simulink model "balancing"  (Simulink 9.1)
settings: Solver=ode1  StartTime=0.0  StopTime=30  FixedStep=0.001  RelTol=1e-8  EnableMultiTasking=on
values from neighbouring files (symbols this model uses):
  A = [0  0    1    0 ... (first row only)    [parameters.m]    (also in parameters_real.m)
  B = (Km/Rm)*B    [parameters.m]    (also in parameters_real.m)
  C = [ 1 0 0 0 ... (first row only)    [parameters.m]    (also in parameters_real.m)
  E0 = 0.05    [parameters.m]    (also in parameters_real.m)
  g = 9.81    [parameters.m]    (also in parameters_real.m)
  J2cap = J2 + m2*(l2^2)    (= 0.0055028)    [parameters.m]    (also in parameters_real.m = 0.006520161)
  K = -lqr(A,B,Q,R)    [parameters.m]    (also in parameters_real.m)
  Km = 0.090    (= 0.09)    [parameters.m]    (also in parameters_real.m)
  l2 = 0.148    [parameters.m]    (also in parameters_real.m = 0.233)
  Lm = 0.005    [parameters.m]    (also in parameters_real.m)
  m2 = 0.075    [parameters.m]    (also in parameters_real.m = 0.049)
  Rm = 7.80    (= 7.8)    [parameters.m]    (also in parameters_real.m)
  w1 = J0cap*J2cap    (= 0.00020550921964)    [parameters.m]    (also in parameters_real.m = J0cap*J2cap)
  w2 = J2cap^2    (= 3.028080784e-05)    [parameters.m]    (also in parameters_real.m = 4.25124994659e-05)
  w3 = -(m2^2)*(L1^2)*(l2^2)    (= -9.52216164e-06)    [parameters.m]    (also in parameters_real.m = -4.08366901448e-06)
  x1 = (-J2cap * b1)    (= -5.5028e-07)    [parameters.m]    (also in parameters_real.m = -6.520161e-07)
  x2 = (m2* L1* l2* b2)    (= 8.64024e-07)    [parameters.m]    (also in parameters_real.m = 5.6582652e-07)
  x3 = - J2cap^2    (= -3.028080784e-05)    [parameters.m]    (also in parameters_real.m = -4.25124994659e-05)
  x4 = - 0.5 *J2cap *m2 *L1* l2    (= -8.49027012e-06)    [parameters.m]    (also in parameters_real.m = -6.58800001512e-06)
  x5 = J2cap *m2*L1*l2    (= 1.698054024e-05)    [parameters.m]    (also in parameters_real.m = 1.31760000302e-05)
  x6 = J2cap    (= 0.0055028)    [parameters.m]    (also in parameters_real.m = 0.006520161)
  x7 = -m2*L1*l2    (= -0.0030858)    [parameters.m]    (also in parameters_real.m = -0.002020809)
  x8 = 0.5* (m2^2)*(L1)*(l2^2)    (= 1.712619e-05)    [parameters.m]    (also in parameters_real.m = 1.15357881765e-05)
  y1 = (m2 * L1 *l2 *b1)    (= 3.0858e-07)    [parameters.m]    (also in parameters_real.m = 2.020809e-07)
  y10 = J2cap    (= 0.0055028)    [parameters.m]    (also in parameters_real.m = 0.006520161)
  y11 = -m2*l2*J0cap    (= -0.00041454393)    [parameters.m]    (also in parameters_real.m = -m2*l2*J0cap)
  y12 = -m2*l2*J2cap    (= -6.108108e-05)    [parameters.m]    (also in parameters_real.m = -7.4440678137e-05)
  y2 = (-J0cap *b2)    (= -1.0456964e-05)    [parameters.m]    (also in parameters_real.m = (-J0cap *b2))
  y3 = -b2* J2cap    (= -1.540784e-06)    [parameters.m]    (also in parameters_real.m = -1.82564508e-06)
  y4 = (m2 * L1* l2 *J2cap)    (= 1.698054024e-05)    [parameters.m]    (also in parameters_real.m = 1.31760000302e-05)
  y5 = 0.5*J0cap* J2cap    (= 0.00010275460982)    [parameters.m]    (also in parameters_real.m = 0.5*J0cap* J2cap)
  y6 = 0.5* J2cap^2    (= 1.514040392e-05)    [parameters.m]    (also in parameters_real.m = 2.1256249733e-05)
  y7 = -0.5 * (m2^2)*(L1^2)*(l2^2)    (= -4.76108082e-06)    [parameters.m]    (also in parameters_real.m = -2.04183450724e-06)
  y8 = -(m2 * L1* l2)    (= -0.0030858)    [parameters.m]    (also in parameters_real.m = -0.002020809)
  y9 = J0cap    (= 0.0373463)    [parameters.m]    (also in parameters_real.m = J0cap)
libraries: simulink_extras x1
settings Model: Creator=mecmg  LastModifiedBy=nhamp
settings DataIOCC: LimitDataPoints=on  SignalLoggingSaveFormat=ModelDataLogs
settings OptimizationCC: ExpressionDepthLimit=2147483647
settings DebuggingCC: SolverPrmCheckMsg=warning  FcnCallInpInsideContextMsg=warning  StateNameClashWarn=warning
settings GRTTargetCC: GeneratePreprocessorConditionals=Disable all

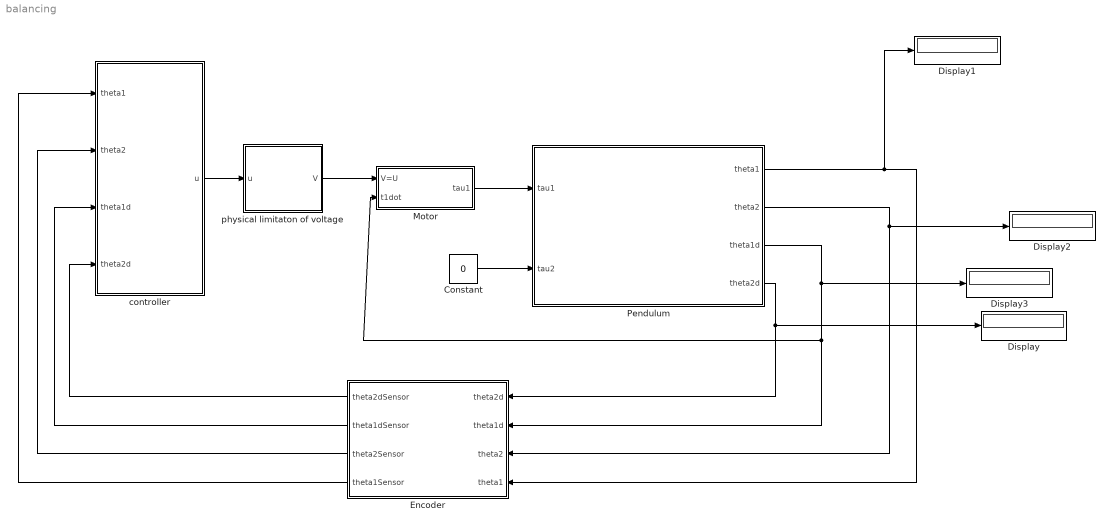
== system balancing ==
  Constant : Constant  Value=0  VectorParams1D=off
  Display{,1..3} (4 alike) : Display
  Encoder : Subsystem
  Motor : Subsystem
  Pendulum : Subsystem
  controller : Subsystem
  physical limitaton of voltage : Subsystem
  wires:
  controller/1(u) -> physical limitaton of voltage/1(u)
  Constant/1 -> Pendulum/2(tau2)
  Pendulum/4(theta2d) -> Encoder/1(theta2d), Display/1
  Encoder/1(theta2dSensor) -> controller/4(theta2d)
  Encoder/4(theta1Sensor) -> controller/1(theta1)
  Encoder/2(theta1dSensor) -> controller/3(theta1d)
  Encoder/3(theta2Sensor) -> controller/2(theta2)
  Motor/1(tau1) -> Pendulum/1(tau1)
  Pendulum/2(theta2) -> Display2/1, Encoder/3(theta2)
  Pendulum/1(theta1) -> Display1/1, Encoder/4(theta1)
  physical limitaton of voltage/1(V) -> Motor/1(V=U)
  Pendulum/3(theta1d) -> Display3/1, Encoder/2(theta1d), Motor/2(t1dot)

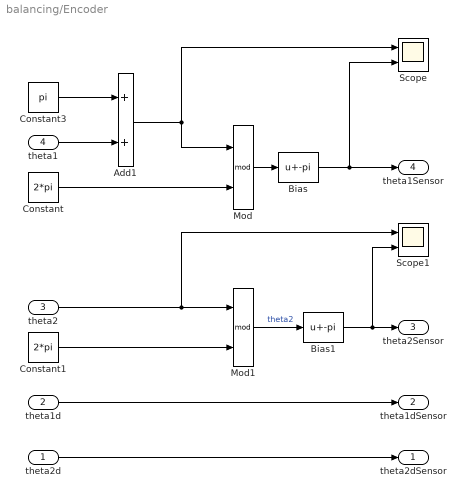
== system balancing/Encoder ==
  theta2d : Inport
  theta1d : Inport  Port=2
  theta2 : Inport  Port=3
  theta1 : Inport  Port=4
  Add1 : Sum
  Bias : Bias  Bias=-pi
  Bias1 : Bias  Bias=-pi
  Constant : Constant  Value=2*pi
  Constant1 : Constant  Value=2*pi
  Constant3 : Constant  Value=pi
  Mod : Math  Operator=mod  SaturateOnIntegerOverflow=on
  Mod1 : Math  Operator=mod  SaturateOnIntegerOverflow=on
  Scope : Scope  NumInputPorts=2
  Scope1 : Scope  NumInputPorts=2
  theta2dSensor : Outport
  theta1dSensor : Outport  Port=2
  theta2Sensor : Outport  Port=3
  theta1Sensor : Outport  Port=4
  wires:
  theta1d/1 -> theta1dSensor/1
  theta2d/1 -> theta2dSensor/1
  Mod1/1 -> Bias1/1  "theta2"
  Constant1/1 -> Mod1/2
  Constant/1 -> Mod/2
  Mod/1 -> Bias/1
  theta2/1 -> Scope1/1, Mod1/1
  theta1/1 -> Add1/2
  Constant3/1 -> Add1/1
  Add1/1 -> Scope/1, Mod/1
  Bias/1 -> Scope/2, theta1Sensor/1
  Bias1/1 -> Scope1/2, theta2Sensor/1

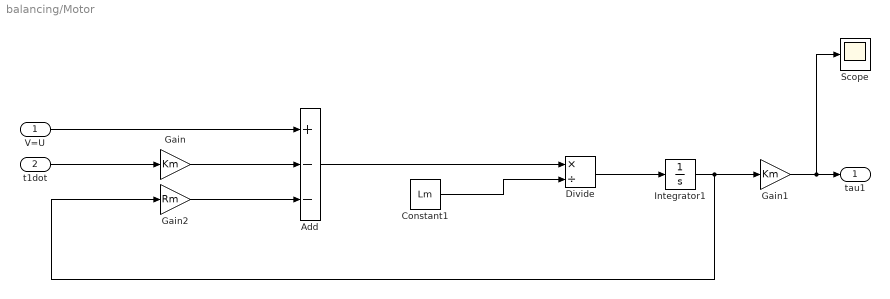
== system balancing/Motor ==
  V=U : Inport
  t1dot : Inport  Port=2
  Add : Sum  Inputs=+--
  Constant1 : Constant  Value=Lm
  Divide : Product  Inputs=*/
  Gain : Gain  Gain=Km
  Gain1 : Gain  Gain=Km
  Gain2 : Gain  Gain=Rm
  Integrator1 : Integrator
  Scope : Scope
  tau1 : Outport
  wires:
  V=U/1 -> Add/1
  t1dot/1 -> Gain/1
  Gain/1 -> Add/2
  Add/1 -> Divide/1
  Constant1/1 -> Divide/2
  Divide/1 -> Integrator1/1
  Integrator1/1 -> Gain2/1, Gain1/1
  Gain1/1 -> Scope/1, tau1/1
  Gain2/1 -> Add/3

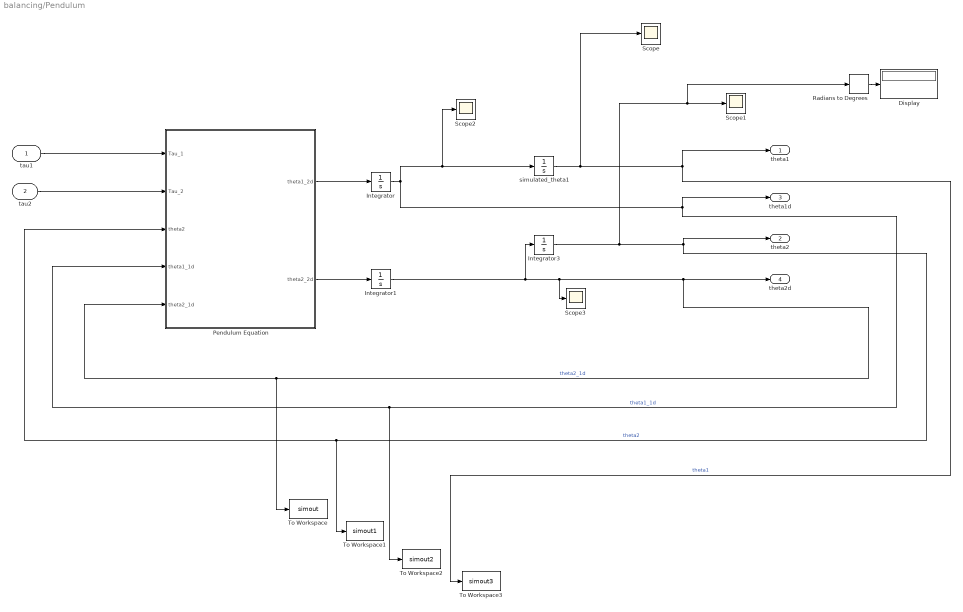
== system balancing/Pendulum ==
  tau1 : Inport
  tau2 : Inport  Port=2
  Display : Display
  Integrator : Integrator
  Integrator1 : Integrator
  Integrator3 : Integrator  InitialCondition=pi-0.085
  Pendulum Equation : Subsystem
  Radians to Degrees : simulink_extras/Transformations/Radians to Degrees
  Scope{,1..3} (4 alike) : Scope
  To Workspace : ToWorkspace  VariableName=simout  SaveFormat=Timeseries  SampleTime=-1
  To Workspace1 : ToWorkspace  VariableName=simout1  SaveFormat=Timeseries  SampleTime=-1
  To Workspace2 : ToWorkspace  VariableName=simout2  SaveFormat=Timeseries  SampleTime=-1
  To Workspace3 : ToWorkspace  VariableName=simout3  SaveFormat=Timeseries  SampleTime=-1
  simulated_theta1 : Integrator
  theta1 : Outport
  theta2 : Outport  Port=2
  theta1d : Outport  Port=3
  theta2d : Outport  Port=4
  wires:
  Pendulum Equation/2(theta2_2d) -> Integrator1/1
  tau2/1 -> Pendulum Equation/2(Tau_2)
  Integrator3/1 -> Scope1/1, Radians to Degrees/1, To Workspace1/1, Pendulum Equation/3(theta2), theta2/1  "theta2"
  simulated_theta1/1 -> Scope/1, To Workspace3/1, theta1/1  "theta1"
  Integrator/1 -> Scope2/1, simulated_theta1/1, To Workspace2/1, Pendulum Equation/4(theta1_1d), theta1d/1  "theta1_1d"
  Integrator1/1 -> Scope3/1, theta2d/1, To Workspace/1, Pendulum Equation/5(theta2_1d), Integrator3/1  "theta2_1d"
  Pendulum Equation/1(theta1_2d) -> Integrator/1
  tau1/1 -> Pendulum Equation/1(Tau_1)
  Radians to Degrees/1 -> Display/1

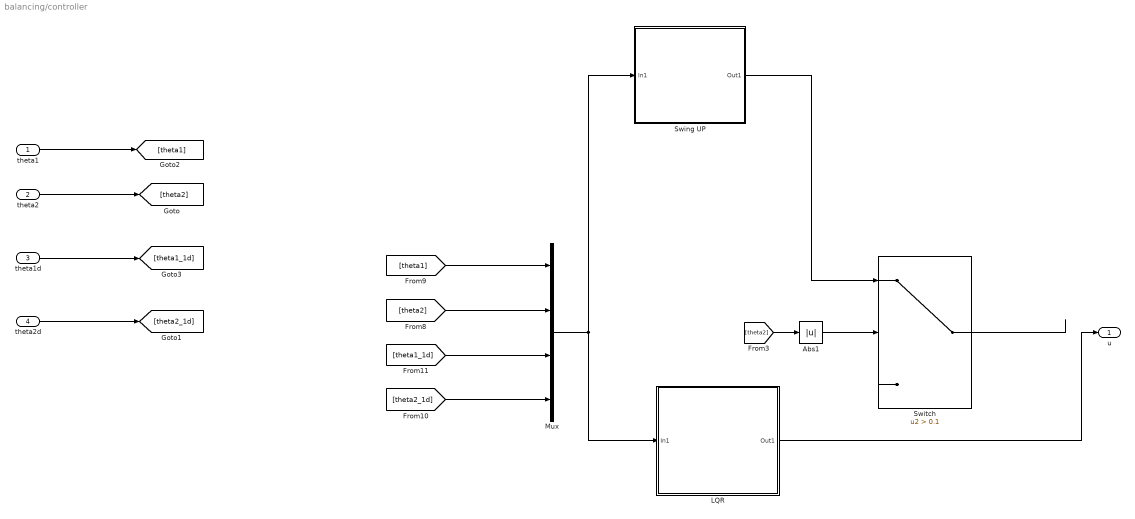
== system balancing/controller ==
  theta1 : Inport
  theta2 : Inport  Port=2
  theta1d : Inport  Port=3
  theta2d : Inport  Port=4
  Abs1 : Abs
  LQR : Subsystem
  Mux : Mux
  Swing UP : Subsystem
  Switch : Switch  Criteria=u2 > Threshold  Threshold=0.1
  u : Outport
  wires:
  theta2/1 -> [theta2]
  theta2d/1 -> [theta2_1d]
  theta1d/1 -> [theta1_1d]
  theta1/1 -> [theta1]
  [theta2] -> Abs1/1
  [theta1] -> Mux/1
  [theta2] -> Mux/2
  [theta1_1d] -> Mux/3
  [theta2_1d] -> Mux/4
  Abs1/1 -> Switch/2
  Mux/1 -> Swing UP/1(In1), LQR/1(In1)
  Switch/1 -> ?
  Swing UP/1(Out1) -> Switch/1
  LQR/1(Out1) -> u/1

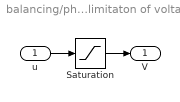
== system balancing/physical limitaton of voltage ==
  u : Inport
  Saturation : Saturate  UpperLimit=10  LowerLimit=-10
  V : Outport
  wires:
  u/1 -> Saturation/1
  Saturation/1 -> V/1

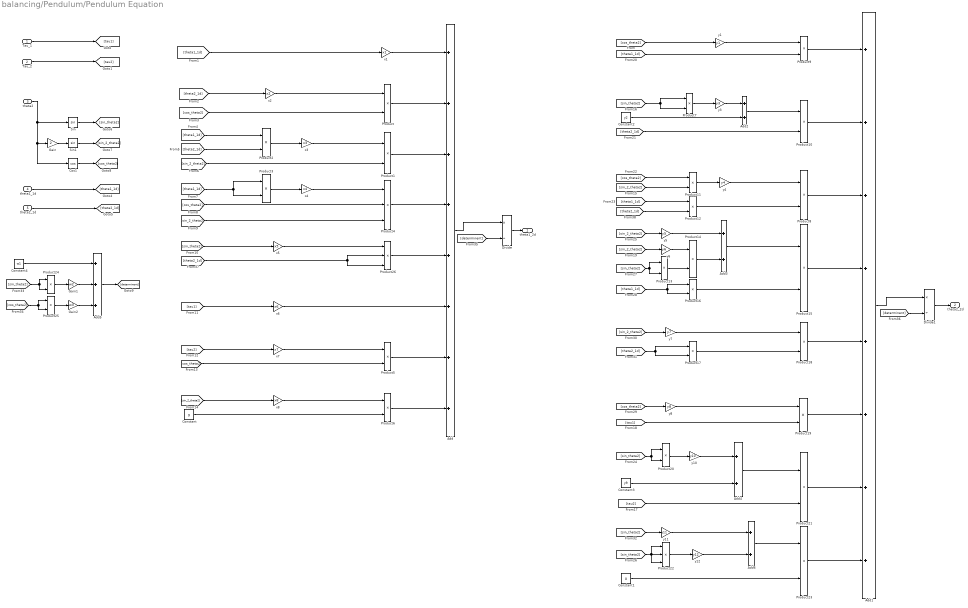
== system balancing/Pendulum/Pendulum Equation ==
  Tau_1 : Inport
  Tau_2 : Inport  Port=2
  theta2 : Inport  Port=3
  theta1_1d : Inport  Port=4
  theta2_1d : Inport  Port=5
  Add : Sum  Inputs=++++++++
  Add1 : Sum  Inputs=++++++++
  Add{2..4,6} (4 alike) : Sum
  Add5 : Sum  Inputs=+++
  Constant : Constant  Value=g
  Constant1 : Constant  Value=g
  Constant2 : Constant  Value=y2
  Constant3 : Constant  Value=y9
  Constant4 : Constant  Value=w1
  Cos1 : Trigonometry  Operator=cos
  Divide : Product  Inputs=*/
  Divide1 : Product  Inputs=*/
  Gain : Gain  Gain=2
  Gain1 : Gain  Gain=w2
  Gain2 : Gain  Gain=w3
  Product{,1..3,5..21,23..25} (24 alike) : Product
  Product22 : Product  Inputs=3
  Product26 : Product  Inputs=3
  Product4 : Product  Inputs=3
  Sin : Trigonometry
  Sin1 : Trigonometry
  x1 : Gain  Gain=x1
  x2 : Gain  Gain=x2
  x3 : Gain  Gain=x3
  x4 : Gain  Gain=x4
  "x5 " : Gain  Gain=x5
  x6 : Gain  Gain=x6
  "x7 " : Gain  Gain=x7
  "x8 " : Gain  Gain=x8
  y1 : Gain  Gain=y1
  y10 : Gain  Gain=y10
  y11 : Gain  Gain=y11
  y12 : Gain  Gain=y12
  y3 : Gain  Gain=y3
  y4 : Gain  Gain=y4
  y5 : Gain  Gain=y5
  y6 : Gain  Gain=y6
  y7 : Gain  Gain=y7
  y8 : Gain  Gain=y8
  theta1_2d : Outport
  theta2_2d : Outport  Port=2
  wires:
  y7/1 -> Product18/1
  y3/1 -> Add2/1
  Constant2/1 -> Add2/2
  y6/1 -> Product14/1
  Product12/1 -> Product8/2
  y5/1 -> Add3/1
  Tau_1/1 -> [tau1]
  Tau_2/1 -> [tau2]
  theta2/1 -> Sin/1, Cos1/1, Gain/1
  theta1_1d/1 -> [theta1_1d]
  theta2_1d/1 -> [theta2_1d]
  Sin/1 -> [sin_theta2]
  Gain/1 -> Sin1/1
  Sin1/1 -> [sin_2_theta2]
  Cos1/1 -> [cos_theta2]
  [theta1_1d] -> x1/1
  x1/1 -> Add/1
  [theta2_1d] -> x2/1
  x2/1 -> Product/1
  Product/1 -> Add/2
  [cos_theta2] -> Product/2
  [theta1_1d] -> Product2/1
  [theta2_1d] -> Product2/2
  Product2/1 -> x3/1
  x3/1 -> Product1/1
  [sin_2_theta2] -> Product1/2
  Product1/1 -> Add/3
  [theta1_1d] -> Product3/2, Product3/1
  Product3/1 -> x4/1
  x4/1 -> Product4/1
  [cos_theta2] -> Product4/2
  [sin_2_theta2] -> Product4/3
  Product4/1 -> Add/4
  [sin_theta2] -> "x5 "/1
  [tau1] -> x6/1
  x6/1 -> Add/6
  [tau2] -> "x7 "/1
  "x7 "/1 -> Product5/1
  [cos_theta2] -> Product5/2
  Product5/1 -> Add/7
  [sin_2_theta2] -> "x8 "/1
  "x8 "/1 -> Product6/1
  Constant/1 -> Product6/2
  Product6/1 -> Add/8
  [cos_theta2] -> y1/1
  [sin_theta2] -> Product7/1, Product7/2
  Product7/1 -> y3/1
  [theta1_1d] -> Product9/2
  y1/1 -> Product9/1
  Product9/1 -> Add1/1
  Product10/1 -> Add1/2
  Add2/1 -> Product10/1
  [theta2_1d] -> Product10/2
  Product8/1 -> Add1/3
  [cos_theta2] -> Product11/1
  [sin_2_theta2] -> Product11/2
  [theta1_1d] -> Product12/1
  [sin_2_theta2] -> y5/1
  [sin_theta2] -> Product13/1, Product13/2
  [sin_2_theta2] -> y6/1
  Product13/1 -> Product14/2
  Product14/1 -> Add3/2
  Add3/1 -> Product15/1
  Product15/1 -> Add1/4
  [theta1_1d] -> Product16/2, Product16/1
  Product16/1 -> Product15/2
  [sin_2_theta2] -> y7/1
  [theta2_1d] -> Product17/1, Product17/2
  Product17/1 -> Product18/2
  Product18/1 -> Add1/5
  [cos_theta2] -> y8/1
  y8/1 -> Product19/1
  [tau1] -> Product19/2
  Product19/1 -> Add1/6
  [sin_theta2] -> Product20/1, Product20/2
  Product20/1 -> y10/1
  y10/1 -> Add4/1
  Constant3/1 -> Add4/2
  Add4/1 -> Product21/1
  [tau2] -> Product21/2
  Product21/1 -> Add1/7
  Product22/1 -> y12/1
  [sin_theta2] -> Product22/1, Product22/3, Product22/2
  [sin_theta2] -> y11/1
  Constant1/1 -> Product23/2
  Product23/1 -> Add1/8
  [sin_theta2] -> Product24/2, Product24/1
  Product24/1 -> Gain1/1
  [cos_theta2] -> Product25/2, Product25/1
  Product25/1 -> Gain2/1
  Constant4/1 -> Add5/1
  Gain1/1 -> Add5/2
  Gain2/1 -> Add5/3
  Add5/1 -> [determinent]
  Add/1 -> Divide/1
  Divide/1 -> theta1_2d/1
  [determinent] -> Divide/2
  Add1/1 -> Divide1/1
  Divide1/1 -> theta2_2d/1
  [determinent] -> Divide1/2
  "x5 "/1 -> Product26/1
  [theta2_1d] -> Product26/3, Product26/2
  Product26/1 -> Add/5
  Product11/1 -> y4/1
  y4/1 -> Product8/1
  [theta2_1d] -> Product12/2
  y12/1 -> Add6/2
  y11/1 -> Add6/1
  Add6/1 -> Product23/1

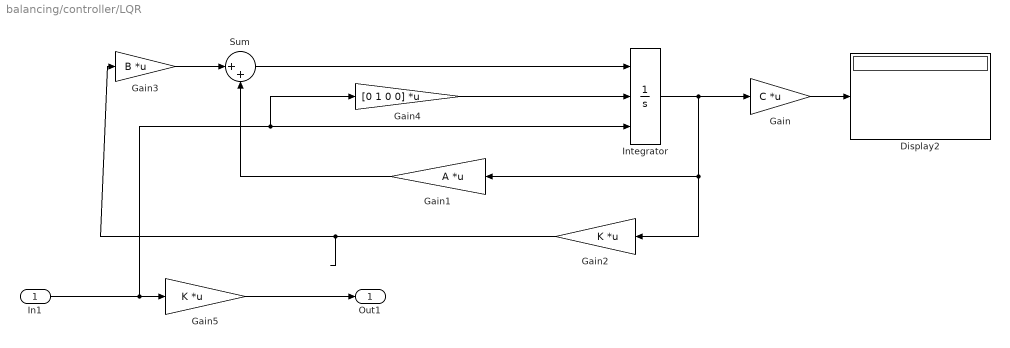
== system balancing/controller/LQR ==
  In1 : Inport
  Display2 : Display
  Gain : Gain  Gain=C  Multiplication=Matrix(K*u)
  Gain1 : Gain  Gain=A  Multiplication=Matrix(K*u)
  Gain2 : Gain  Gain=K  Multiplication=Matrix(K*u)
  Gain3 : Gain  Gain=B  Multiplication=Matrix(K*u)
  Gain4 : Gain  Gain=[0 1 0 0]  Multiplication=Matrix(K*u)
  Gain5 : Gain  Gain=K  Multiplication=Matrix(K*u)
  Integrator : Integrator  ExternalReset=rising  InitialConditionSource=external
  Sum : Sum  Inputs=|++
  Out1 : Outport
  wires:
  Gain/1 -> Display2/1
  Gain3/1 -> Sum/1
  Integrator/1 -> Gain2/1, Gain1/1, Gain/1
  Gain1/1 -> Sum/2
  Sum/1 -> Integrator/1
  Gain2/1 -> Gain3/1
  Gain4/1 -> Integrator/2
  Gain5/1 -> Out1/1
  In1/1 -> Gain4/1, Integrator/3, Gain5/1

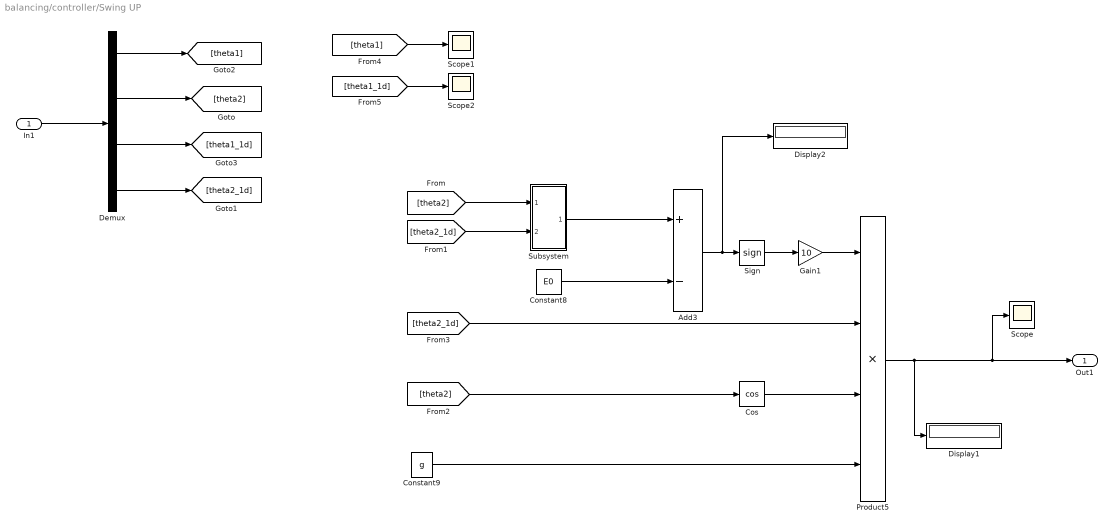
== system balancing/controller/Swing UP ==
  In1 : Inport
  Add3 : Sum  Inputs=+-
  Constant8 : Constant  Value=E0
  Constant9 : Constant  Value=g
  Cos : Trigonometry  Operator=cos
  Demux : Demux
  Display1 : Display
  Display2 : Display
  Gain1 : Gain  Gain=10
  Product5 : Product  Inputs=4
  Scope : Scope
  Scope1 : Scope
  Scope2 : Scope
  Sign : Signum
  Subsystem : Subsystem
  Out1 : Outport
  wires:
  Add3/1 -> Display2/1, Sign/1
  Cos/1 -> Product5/3
  Subsystem/1(Out1) -> Add3/1
  Constant9/1 -> Product5/4
  Sign/1 -> Gain1/1
  Constant8/1 -> Add3/2
  Gain1/1 -> Product5/1
  [theta2] -> Cos/1
  [theta2_1d] -> Product5/2
  In1/1 -> Demux/1
  Demux/1 -> [theta1]
  Demux/3 -> [theta1_1d]
  Demux/4 -> [theta2_1d]
  [theta2] -> Subsystem/1(In1)
  [theta2_1d] -> Subsystem/2(In2)
  Product5/1 -> Scope/1, Out1/1, Display1/1
  [theta1] -> Scope1/1
  [theta1_1d] -> Scope2/1
  Demux/2 -> [theta2]

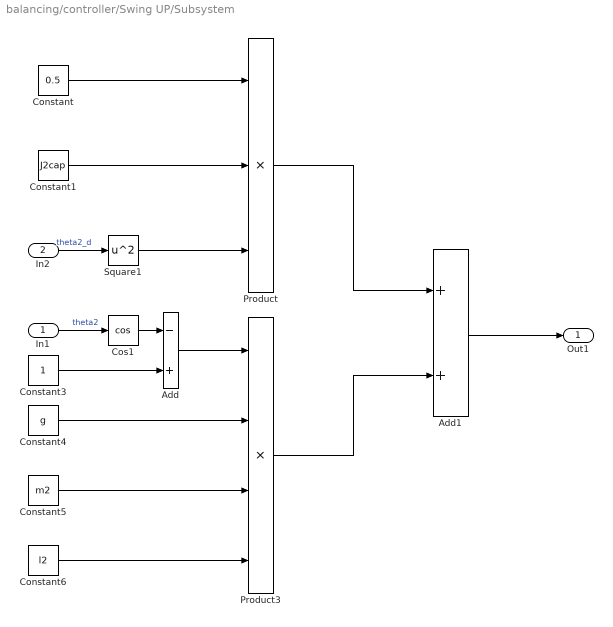
== system balancing/controller/Swing UP/Subsystem ==
  In1 : Inport
  In2 : Inport  Port=2
  Add : Sum  Inputs=-+
  Add1 : Sum
  Constant : Constant  Value=0.5
  Constant1 : Constant  Value=J2cap
  Constant3 : Constant
  Constant4 : Constant  Value=g
  Constant5 : Constant  Value=m2
  Constant6 : Constant  Value=l2
  Cos1 : Trigonometry  Operator=cos
  Product : Product  Inputs=3
  Product3 : Product  Inputs=4
  Square1 : Math  Operator=square  SaturateOnIntegerOverflow=on
  Out1 : Outport
  wires:
  Add/1 -> Product3/1
  Cos1/1 -> Add/1
  Constant3/1 -> Add/2
  Constant4/1 -> Product3/2
  Constant1/1 -> Product/2
  Square1/1 -> Product/3
  Constant5/1 -> Product3/3
  Constant/1 -> Product/1
  Constant6/1 -> Product3/4
  Product3/1 -> Add1/2
  Product/1 -> Add1/1
  Add1/1 -> Out1/1
  In1/1 -> Cos1/1  "theta2"
  In2/1 -> Square1/1  "theta2_d"
